simulink model "ex6_a"  (R2020a)
settings: Solver=VariableStepAuto  StartTime=0.0  StopTime=3e6  RelTol=1e-3
settings Model: Creator=반달  LastModifiedBy=반달

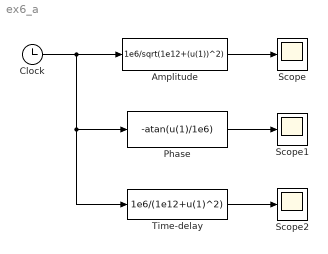
== system ex6_a ==
  Amplitude : Fcn  Expr=1e6/sqrt(1e12+(u(1))^2)
  Clock : Clock
  Phase : Fcn  Expr=-atan(u(1)/1e6)
  Scope : Scope
  Scope1 : Scope
  Scope2 : Scope
  Time-delay : Fcn  Expr=1e6/(1e12+u(1)^2)
  wires:
  Clock/1 -> Time-delay/1, Phase/1, Amplitude/1
  Phase/1 -> Scope1/1
  Amplitude/1 -> Scope/1
  Time-delay/1 -> Scope2/1
